simulink model "carPlant_smoothUp_followerStopper"  (R2018b)
settings: Solver=VariableStepAuto  StartTime=0.0  StopTime=inf  RelTol=1e-3
undefined symbols (not defined in the file or in its folder): Angular, Linear
libraries: robotlib x5, autolibshared x2
settings Model: Creator=ckreienk  LastModifiedBy=ckreienk

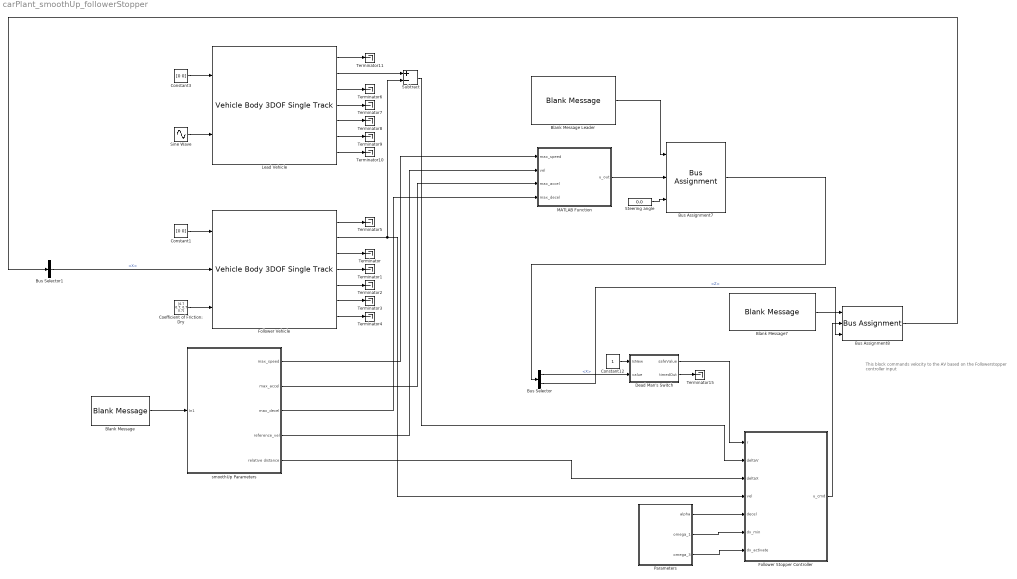
== system carPlant_smoothUp_followerStopper ==
  note: This block commands velocity to the AV based
      | on the Followerstopper controller input
  Blank Message : robotlib/Blank Message  messageClass=Message  entityType=geometry_msgs/Point  messageType=geometry_msgs/Point  SampleTime=inf
      settings: SourceProductBaseCode=RO
  Blank Message Leader : robotlib/Blank Message  messageClass=Message  entityType=geometry_msgs/Twist  messageType=geometry_msgs/Twist  SampleTime=inf
      settings: SourceProductBaseCode=RO
  Blank Message7 : robotlib/Blank Message  messageClass=Message  entityType=geometry_msgs/Twist  messageType=geometry_msgs/Twist  SampleTime=inf
      settings: SourceProductBaseCode=RO
  Bus Assignment7 : BusAssignment  AssignedSignals=Linear.X,Angular.Z
  Bus Assignment8 : BusAssignment  AssignedSignals=Linear.X,Angular.Z
  Bus Selector : BusSelector  OutputSignals=Linear.X,Angular.Z
  Bus Selector1 : BusSelector  OutputSignals=Linear.X
  Coefficient of Friction: Dry : Constant  Value=[0.7 0.7; 0.7 0.7]
  Constant1 : Constant  Value=[0 0]
  Constant12 : Constant
  Constant3 : Constant  Value=[0 0]
  Dead Man's Switch : Subsystem  TreatAsAtomicUnit=on  mask{stepSize=0.05, timeout=0.2}
      mask prompts: stepSize "Simulation step size"; timeout "Timeout (in seconds)"
      mask help: Interprets whether a new message has been recently received, and if so permits the data in 'value' to be passed through. Otherwise, 0 is outputted from 'safeValue'
      mask Help: Interprets whether a new message has been recently received, and if so permits the data in 'value' to be passed through. Otherwise, 0 is outputted from 'safeValue'
  Follower Stopper Controller : Subsystem
  Follower Vehicle : autolibshared/Vehicle Body 3DOF Single Track  trackMode=Dual  inputMode=External longitudinal velocity  frontSteerMode=on  rearSteerMode=off  windMode=off  muMode=on  extFMode=off  extMMode=off  aMode=2  NF=2  NR=2  m=2000  a=1.4  b=1.6  h=0.35  X_o=0  xdot_o=0  CalphaMode=off  sigmaMode=on  d=0  w=[1.4,1.4]  Cy_f=12e3  Cy_r=11e3  sigma_f=.1  sigma_r=.1  alpha_f_brk=[-.1 .1]  Cy_f_data=[-9e3 9e3]  alpha_r_brk=[-.1 .1]  Cy_r_data=[-9e3 9e3]  Y_o=0  ydot_o=0  Izz=4000  psi_o=0  r_o=0  Af=2  Cd=.3  Cl=.1  Cpm=.1  beta_w=[0:0.01:0.3]  Cs=[0:0.03:0.9]  Cym=[0:0.01:0.3]  Pabs=101325  Tair=273  g=9.81  mu=1  xdot_tol=.01  Fznom=5000  Fxtire_sat=7e4  Fytire_sat=7e4  longOff=0  latOff=0  vertOff=0
      settings: SourceProductName=Powertrain Blockset  SourceProductBaseCode=PW
  Lead Vehicle : autolibshared/Vehicle Body 3DOF Single Track  trackMode=Dual  inputMode=External longitudinal velocity  frontSteerMode=on  rearSteerMode=off  windMode=off  muMode=off  extFMode=off  extMMode=off  aMode=2  NF=2  NR=2  m=2000  a=1.4  b=1.6  h=0.35  X_o=0  xdot_o=0  CalphaMode=off  sigmaMode=on  d=0  w=[1.4,1.4]  Cy_f=12e3  Cy_r=11e3  sigma_f=.1  sigma_r=.1  alpha_f_brk=[-.1 .1]  Cy_f_data=[-9e3 9e3]  alpha_r_brk=[-.1 .1]  Cy_r_data=[-9e3 9e3]  Y_o=0  ydot_o=0  Izz=4000  psi_o=0  r_o=0  Af=2  Cd=.3  Cl=.1  Cpm=.1  beta_w=[0:0.01:0.3]  Cs=[0:0.03:0.9]  Cym=[0:0.01:0.3]  Pabs=101325  Tair=273  g=9.81  mu=1  xdot_tol=.01  Fznom=5000  Fxtire_sat=7e4  Fytire_sat=7e4  longOff=0  latOff=0  vertOff=0
      settings: SourceProductName=Powertrain Blockset  SourceProductBaseCode=PW
  MATLAB Function : MATLAB Function  TreatAsAtomicUnit=on
  Parameters : Subsystem
  Sine Wave : Sin  Amplitude=20  Bias=20  SampleTime=0
  Steering angle : Constant  Value=0.0
  Subtract : Sum  Inputs=+-
  Terminator{,1..11,15} (13 alike) : Terminator
  smoothUp Parameters : Subsystem
  wires:
  Lead Vehicle/2 -> Subtract/1
  Sine Wave/1 -> Lead Vehicle/2
  Constant3/1 -> Lead Vehicle/1
  Lead Vehicle/7 -> Terminator10/1
  Lead Vehicle/6 -> Terminator9/1
  Lead Vehicle/5 -> Terminator8/1
  Lead Vehicle/4 -> Terminator7/1
  Lead Vehicle/3 -> Terminator6/1
  Lead Vehicle/1 -> Terminator11/1
  Follower Vehicle/1 -> Terminator5/1
  Follower Vehicle/3 -> Terminator/1
  Follower Vehicle/4 -> Terminator1/1
  Follower Vehicle/5 -> Terminator2/1
  Follower Vehicle/6 -> Terminator3/1
  Follower Vehicle/7 -> Terminator4/1
  Constant1/1 -> Follower Vehicle/1
  MATLAB Function/1(u_out) -> Bus Assignment7/2
  Steering angle/1 -> Bus Assignment7/3
  Blank Message Leader/1 -> Bus Assignment7/1
  Parameters/3(omega_3) -> Follower Stopper Controller/7(dx_activate)
  Parameters/2(omega_1) -> Follower Stopper Controller/6(dx_min)
  Parameters/1(alpha) -> Follower Stopper Controller/5(decel)
  Bus Selector/2 -> Bus Assignment8/3  "<Z>"
  Follower Vehicle/2 -> Follower Stopper Controller/4(vel), Subtract/2
  Subtract/1 -> Follower Stopper Controller/2(deltaV)
  Dead Man's Switch/2(timedOut) -> Terminator15/1
  Bus Selector/1 -> Dead Man's Switch/2(value)  "<X>"
  Dead Man's Switch/1(safeValue) -> Follower Stopper Controller/1(r)
  Follower Stopper Controller/1(u_cmd) -> Bus Assignment8/2
  Blank Message7/1 -> Bus Assignment8/1
  Bus Assignment7/1 -> Bus Selector/1
  Constant12/1 -> Dead Man's Switch/1(IsNew)
  Blank Message/1 -> smoothUp Parameters/1(In1)
  Bus Assignment8/1 -> Bus Selector1/1
  smoothUp Parameters/1(max_speed) -> MATLAB Function/1(max_speed)
  smoothUp Parameters/2(max_accel) -> MATLAB Function/3(max_accel)
  smoothUp Parameters/3(max_decel) -> MATLAB Function/4(max_decel)
  smoothUp Parameters/4(reference_vel) -> MATLAB Function/2(vel)
  smoothUp Parameters/5(relative distance) -> Follower Stopper Controller/3(deltaX)
  Bus Selector1/1 -> Follower Vehicle/2  "<X>"
  Coefficient of Friction: Dry/1 -> Follower Vehicle/3

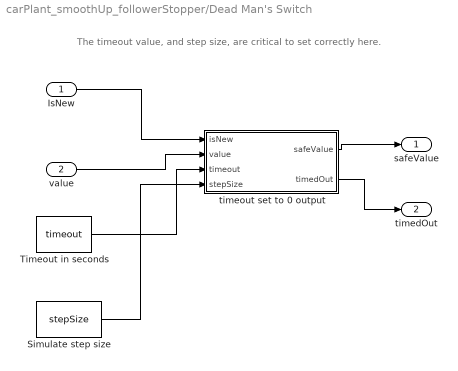
== system carPlant_smoothUp_followerStopper/Dead Man's Switch ==
  note: The timeout value, and step size, are critical to set correctly here.
  IsNew : Inport
  value : Inport  Port=2
  Simulate step size : Constant  Value=stepSize
  Timeout in seconds : Constant  Value=timeout
  timeout set to 0 output : MATLAB Function  TreatAsAtomicUnit=on
  safeValue : Outport  InitialOutput=[0]
  timedOut : Outport  Port=2  InitialOutput=[0]
  wires:
  Simulate step size/1 -> timeout set to 0 output/4(stepSize)
  timeout set to 0 output/2(timedOut) -> timedOut/1
  Timeout in seconds/1 -> timeout set to 0 output/3(timeout)
  value/1 -> timeout set to 0 output/2(value)
  timeout set to 0 output/1(safeValue) -> safeValue/1
  IsNew/1 -> timeout set to 0 output/1(isNew)

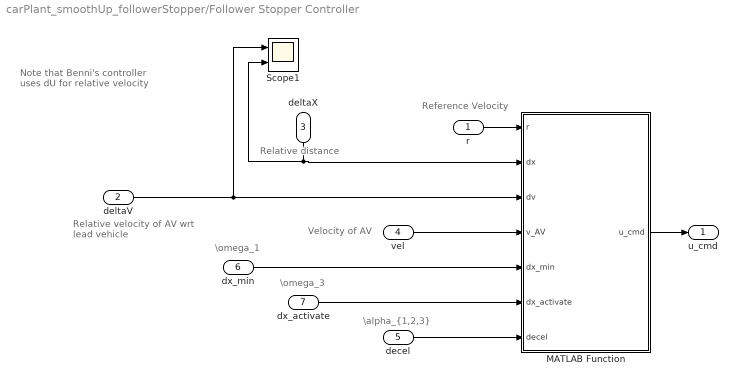
== system carPlant_smoothUp_followerStopper/Follower Stopper Controller ==
  note: \alpha_{1,2,3}
  note: \omega_3
  note: \omega_1
  note: Relative distance
  note: Reference Velocity
  note: Velocity of AV
  note: Relative velocity of
      | AV wrt lead vehicle
  note: Note that Benni's
      | controller uses dU
      | for relative
      | velocity
  r : Inport
  deltaV : Inport  Port=2
  deltaX : Inport  Port=3
  vel : Inport  Port=4
  decel : Inport  Port=5
  dx_min : Inport  Port=6
  dx_activate : Inport  Port=7
  MATLAB Function : MATLAB Function  TreatAsAtomicUnit=on
  Scope1 : Scope  NumInputPorts=2
  u_cmd : Outport
  wires:
  r/1 -> MATLAB Function/1(r)
  dx_activate/1 -> MATLAB Function/6(dx_activate)
  decel/1 -> MATLAB Function/7(decel)
  dx_min/1 -> MATLAB Function/5(dx_min)
  vel/1 -> MATLAB Function/4(v_AV)
  MATLAB Function/1(u_cmd) -> u_cmd/1
  deltaV/1 -> Scope1/1, MATLAB Function/3(dv)
  deltaX/1 -> Scope1/2, MATLAB Function/2(dx)

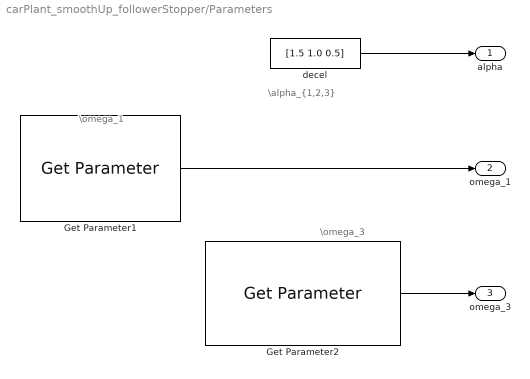
== system carPlant_smoothUp_followerStopper/Parameters ==
  note: \alpha_{1,2,3}
  note: \omega_1
  note: \omega_3
  Get Parameter1 : robotlib/Get Parameter  ParameterSource=Specify your own  ParameterName=/dx_min  ParameterType=double  ParameterMaxArrayLength=16  ParameterInitialValue=4.5  SampleTime=-1  ShowErrorCodeOutput=off  ModelName=carPlant_smoothUp_followerStopper  BlockId=ParamGet_carPlant_smoothUp_followerStopper_99
      settings: SourceProductName=Robotics System Toolbox  SourceProductBaseCode=RO
  Get Parameter2 : robotlib/Get Parameter  ParameterSource=Specify your own  ParameterName=/dx_activate  ParameterType=double  ParameterMaxArrayLength=16  ParameterInitialValue=6.0  SampleTime=-1  ShowErrorCodeOutput=off  ModelName=carPlant_smoothUp_followerStopper  BlockId=ParamGet_carPlant_smoothUp_followerStopper_100
      settings: SourceProductName=Robotics System Toolbox  SourceProductBaseCode=RO
  decel : Constant  Value=[1.5 1.0 0.5]  OutDataTypeStr=double  SampleTime=-1
  alpha : Outport
  omega_1 : Outport  Port=2
  omega_3 : Outport  Port=3
  wires:
  decel/1 -> alpha/1
  Get Parameter1/1 -> omega_1/1
  Get Parameter2/1 -> omega_3/1

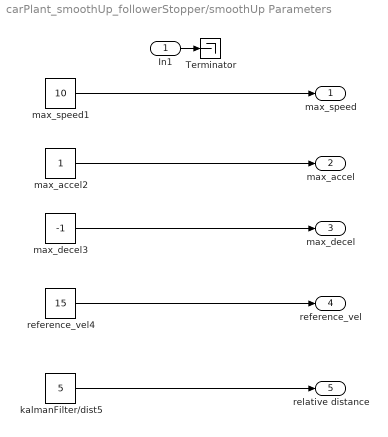
== system carPlant_smoothUp_followerStopper/smoothUp Parameters ==
  In1 : Inport
  Terminator : Terminator
  kalmanFilter/dist5 : Constant  Value=5
  max_accel2 : Constant
  max_decel3 : Constant  Value=-1
  max_speed1 : Constant  Value=10
  reference_vel4 : Constant  Value=15
  max_speed : Outport  Tag=max_speed
  max_accel : Outport  Port=2
  max_decel : Outport  Port=3
  reference_vel : Outport  Port=4
  relative distance : Outport  Port=5
  wires:
  kalmanFilter/dist5/1 -> relative distance/1
  In1/1 -> Terminator/1
  max_speed1/1 -> max_speed/1
  max_accel2/1 -> max_accel/1
  max_decel3/1 -> max_decel/1
  reference_vel4/1 -> reference_vel/1

== matlab function carPlant_smoothUp_followerStopper/Dead Man's Switch/timeout set to 0 output ==
  data: isNew input; safeValue output; value input; timeout input; timedOut output; stepSize input
function [safeValue,timedOut] = fcn(isNew,value,timeout,stepSize)
%#codegen
persistent sinceLastMsg
timedOut=true;
if isempty(sinceLastMsg)
    sinceLastMsg=(timeout/stepSize)+1;
end

safeValue=0;
% if no new message
% after timeout, we output 0
if( isNew == true )
    sinceLastMsg = 0;
else
    sinceLastMsg = sinceLastMsg+1;
end

% Note: we require step size as an input here, and depend on our
% system being executed at a regular rate, or bad things will happen
if( sinceLastMsg < timeout/stepSize )
    timedOut = false;
end
    
if( timedOut == false )
    safeValue = value;
end

== matlab function carPlant_smoothUp_followerStopper/MATLAB Function ==
  data: max_speed input; u_out output; vel input; max_accel input; max_decel input
function u_out = fcn(max_speed,vel,max_accel,max_decel)
%#codegen
persistent y

if isempty(y)
    y=0;
end

% JMS: HACK timestep hacked at 0.05
dt=0.05;
if( y > max_speed + 1 )
    y = max(max_speed,y - abs(max_decel)*dt);
elseif( y < max_speed - 1)
    y = min(max_speed,y + max_accel*dt);
else
    y = double(max_speed);
end

if (y < 2 && max_speed > 2)
    y = 2;
elseif(y < 1 && max_speed > 1)
    y = 1;
end

u_out =min(max(y,vel-1.0),vel+2.0);

== matlab function carPlant_smoothUp_followerStopper/Follower Stopper Controller/MATLAB Function ==
  data: r input; u_cmd output; dx input; dv input; v_AV input; dx_min input; dx_activate input; decel input
function u_cmd = fcn(r,dx,dv,v_AV,...
    dx_min,dx_activate,decel)
%#codegen
% Safety controller, based on quadratic bands.
% Input: r = desired velocity (from other models)
%          dx = estimate of gap to vehicle ahead
%          dv = estimate of time derivative of dx (= velocity difference)
%         v_AV = velocity of AV
%      dx_min = minimum distance
% dx_activate = distance below which controller does something
%       decel = vector of three deceleration values for parabolas
% Out:  u_cmd = actual velocity commanded (always u_cmd<=U)
%
% Controller-specific parameters
dx_mid = (dx_min+dx_activate)/2; % mid distance, where v_lead is commanded
% Lead vehicle velocity
v_lead = v_AV+dv; % velocity of lead vehicle
v_lead = max(v_lead,0); % lead vehicle cannot go backwards
v = min(r,v_lead); % safety velocity cannot exceed desired velocity U
% Treatment of positive dv-values
dv = min(dv,0); % domains for dv>0 same as dv=0
% For given dv, dx-values of band boundaries
dx1 = dx_min+1/(2*decel(1))*dv.^2;
dx2 = dx_mid+1/(2*decel(2))*dv.^2;
dx3 = dx_activate+1/(2*decel(3))*dv.^2;
% Actual commanded velocity
u_cmd = double((dx1<dx&dx<=dx2).*(v.*(dx-dx1)./(dx2-dx1))+...
    (dx2<dx&dx<=dx3).*(v+(r-v).*(dx-dx2)./(dx3-dx2))+...
    (dx3<dx).*r);
% DO not move if within dx_min
% if(dx < dx_min)
%     u_cmd = 0;
% end

if( dx > 16.0 )
    u_cmd = r;
end
